simulink model "HelloWorld"  (R2014a)
settings: Solver=FixedStepDiscrete  StartTime=0.0  StopTime=5  FixedStep=0.01  RelTol=1e-3  SampleTimeConstraint=Specified
libraries: simulink x1, linuxlib x1
settings Model: Creator=ses  LastModifiedBy=ses
settings OptimizationCC: OptimizeModelRefInitCode=on  LifeSpan=1  MaxStackSize=64
settings HardwareCC: ProdLargestAtomicInteger=Long  ProdLargestAtomicFloat=Double  ProdEndianess=LittleEndian  ProdHWDeviceType=ARM Compatible->ARM Cortex
settings RTWCC: SystemTargetFile=ert_linux.tlc  MakeCommand=make_rtw CC=arm-linux-gnueabihf-gcc  TemplateMakefile=ert_linux.tmf  Description=Linux Embedded Coder  ProcessScript=ert_linux_make_rtw_hook  Toolchain=Linaro Toolchain v4.8
settings CodeAppCC: IgnoreCustomStorageClasses=off
settings STFCustomTargetCC: ModelReferenceCompliant=off  ConcurrentExecutionCompliant=off  GeneratePreprocessorConditionals=Use local settings  CombineOutputUpdateFcns=on  ERTCustomFileBanners=on  SupportContinuousTime=off  MATLABClassNameForMDSCustomization=Simulink.SoftwareTarget.ERTCustomization  GRTInterface=off  SystemTargetFile=ert_linux.tlc
settings ERTTargetCC: GenerateSampleERTMain=off  ModelReferenceCompliant=off  SupportNonInlinedSFcns=on  ERTCustomFileTemplate=ert_linux_file_process.tlc

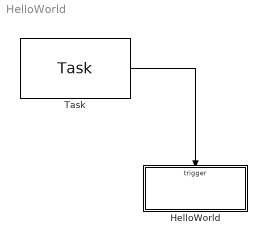
== system HelloWorld ==
  HelloWorld : Subsystem  TreatAsAtomicUnit=on
  Task : linuxlib/Task  taskName=Hello  taskPolicy=SCHED_FIFO  taskPriority=1
  wires:
  Task/1 -> HelloWorld/Trigger

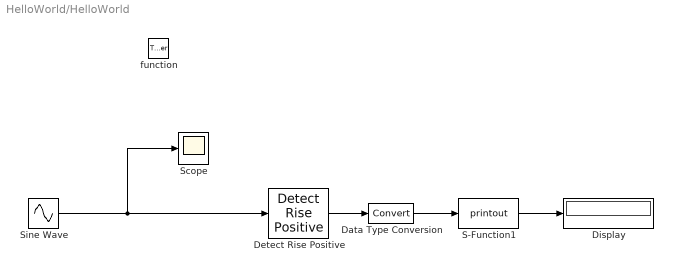
== system HelloWorld/HelloWorld ==
  function : TriggerPort  TriggerType=function-call  SampleTime=0.01
  Data Type Conversion : DataTypeConversion
  Detect Rise Positive : simulink/Logic and Bit Operations/Detect Rise Positive  vinit=0  InputProcessing=Inherited  OutDataTypeStr=boolean
  Display : Display
  S-Function1 : S-Function  FunctionName=printout  EnableBusSupport=off
  Scope : Scope
  Sine Wave : Sin  Frequency=2  Phase=-pi/8
  wires:
  Sine Wave/1 -> Detect Rise Positive/1, Scope/1
  Detect Rise Positive/1 -> Data Type Conversion/1
  S-Function1/1 -> Display/1
  Data Type Conversion/1 -> S-Function1/1
